simulink model "simulacao_sem_linearizar_prbs"  (R2017a)
settings: Solver=VariableStepAuto  StartTime=0.0  StopTime=180  RelTol=1e-3
values from neighbouring files (symbols this model uses):
  a = -9128    [prepare_y_prbs.m]
undefined symbols (not defined in the file or in its folder): g, m
libraries: simulink x1
settings Model: Creator=Mateus  LastModifiedBy=mateu

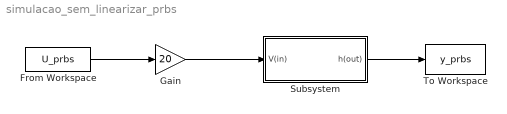
== system simulacao_sem_linearizar_prbs ==
  From Workspace : FromWorkspace  VariableName=U_prbs  SampleTime=0.1  Interpolate=off  OutputAfterFinalValue=Setting to zero
  Gain : Gain  Gain=20
  Subsystem : Subsystem
  To Workspace : ToWorkspace  VariableName=y_prbs  SaveFormat=Timeseries  SampleTime=0.1
  wires:
  Subsystem/1(h(out)) -> To Workspace/1
  Gain/1 -> Subsystem/1(V(in))
  From Workspace/1 -> Gain/1

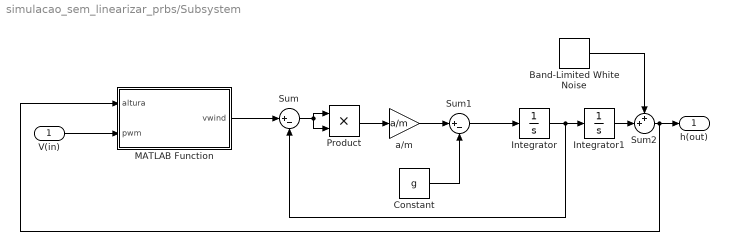
== system simulacao_sem_linearizar_prbs/Subsystem ==
  V(in) : Inport
  Band-Limited White Noise : simulink/Sources/Band-Limited White Noise  Cov=[0.03]  Ts=0.1  seed=[23341]
  Constant : Constant  Value=g
  Integrator : Integrator
  Integrator1 : Integrator  InitialCondition=0.2
  MATLAB Function : MATLAB Function  TreatAsAtomicUnit=on
  Product : Product
  Sum : Sum  Inputs=|+-
  Sum1 : Sum  Inputs=|+-
  Sum2 : Sum  Inputs=++|
  a/m : Gain  Gain=a/m
  h(out) : Outport
  wires:
  Sum2/1 -> h(out)/1, MATLAB Function/1(altura)
  MATLAB Function/1(vwind) -> Sum/1
  Band-Limited White Noise/1 -> Sum2/1
  Sum/1 -> Product/1, Product/2
  a/m/1 -> Sum1/1
  V(in)/1 -> MATLAB Function/2(pwm)
  Constant/1 -> Sum1/2
  Sum1/1 -> Integrator/1
  Product/1 -> a/m/1
  Integrator1/1 -> Sum2/2
  Integrator/1 -> Sum/2, Integrator1/1

== matlab function simulacao_sem_linearizar_prbs/Subsystem/MATLAB Function ==
  data: altura input; vwind output; pwm input
function vwind = fittedmodel(altura,pwm)

p00 =       18.37;
p10 =     -0.5502;
p01 =       0.224;
p20 =      0.0105;
p11 =   -0.003002;
p02 =  -0.0006906;
p30 =  -6.885e-05;
p21 =   1.084e-05;
p12 =   8.743e-06;
p03 =   2.752e-07;
vwind = p00 + p10*altura + p01*pwm + p20*altura^2 + p11*altura*pwm + p02*pwm^2 + p30*altura^3 + p21*altura^2*pwm + p12*altura*pwm^2 + p03*pwm^3;
if vwind <0 
    vwind=0;
end

end
